simulink model "AirplaneSimModel_Trim"  (R2025b)
settings: Solver=ode1  StartTime=0.0  StopTime=1  RelTol=1e-3
model workspace (MAT data in the model file):
  initial_input_in_model_workspace = [0 0.010416783094 0.861959012587 0.2094 -0.018208861967 0.815245721637]
  initial_state_in_model_workspace.time = 0
  initial_state_in_model_workspace.signals(1).values = [0 0 0]
  initial_state_in_model_workspace.signals(1).dimensions = 3
  initial_state_in_model_workspace.signals(1).label = 'CSTATE'
  initial_state_in_model_workspace.signals(1).blockName = 'AirplaneSimModel_Trim/Conventional Airplane,
    | single engine/State equations
    | (Quaternions)/s__g'
  initial_state_in_model_workspace.signals(1).stateName = 'position'
  initial_state_in_model_workspace.signals(1).inReferencedModel = 0
  initial_state_in_model_workspace.signals(1).sampleTime = [0 0]
  initial_state_in_model_workspace.signals(2).values = [0.9988 0 -0.125422444495 0]
  initial_state_in_model_workspace.signals(2).dimensions = 4
  initial_state_in_model_workspace.signals(2).label = 'CSTATE'
  initial_state_in_model_workspace.signals(2).blockName = 'AirplaneSimModel_Trim/Conventional Airplane,
    | single engine/State equations
    | (Quaternions)/q_bg'
  initial_state_in_model_workspace.signals(2).stateName = 'quaternion'
  initial_state_in_model_workspace.signals(2).inReferencedModel = 0
  initial_state_in_model_workspace.signals(2).sampleTime = [0 0]
  initial_state_in_model_workspace.signals(3).values = 797.872042942
  initial_state_in_model_workspace.signals(3).dimensions = 1
  initial_state_in_model_workspace.signals(3).label = 'CSTATE'
  initial_state_in_model_workspace.signals(3).blockName = 'AirplaneSimModel_Trim/Conventional Airplane,
    | single engine/Actuators/Integrator'
  initial_state_in_model_workspace.signals(3).stateName = 'motor_speed'
  initial_state_in_model_workspace.signals(3).inReferencedModel = 0
  initial_state_in_model_workspace.signals(3).sampleTime = [0 0]
  initial_state_in_model_workspace.signals(4).values = 0.0767491085272
  initial_state_in_model_workspace.signals(4).dimensions = 1
  initial_state_in_model_workspace.signals(4).label = 'CSTATE'
  initial_state_in_model_workspace.signals(4).blockName = 'AirplaneSimModel_Trim/Conventional Airplane,
    | single engine/Actuators/Nonlinear Second-Order Actuator
    | (elevons)/A'
  initial_state_in_model_workspace.signals(4).stateName = 'A'
  initial_state_in_model_workspace.signals(4).inReferencedModel = 0
  initial_state_in_model_workspace.signals(4).sampleTime = [0 0]
  initial_state_in_model_workspace.signals(5).values = 0.0434586983747
  initial_state_in_model_workspace.signals(5).dimensions = 1
  initial_state_in_model_workspace.signals(5).label = 'CSTATE'
  initial_state_in_model_workspace.signals(5).blockName = 'AirplaneSimModel_Trim/Conventional Airplane,
    | single engine/Actuators/Nonlinear Second-Order Actuator
    | (htpTrim)/A'
  initial_state_in_model_workspace.signals(5).stateName = 'A'
  initial_state_in_model_workspace.signals(5).inReferencedModel = 0
  initial_state_in_model_workspace.signals(5).sampleTime = [0 0]
  initial_state_in_model_workspace.signals(6).values = [0.426323238582 0.426323238582 0.416142037484 0.416142037484]
  initial_state_in_model_workspace.signals(6).dimensions = 4
  initial_state_in_model_workspace.signals(6).label = 'CSTATE'
  initial_state_in_model_workspace.signals(6).blockName = 'AirplaneSimModel_Trim/Conventional Airplane,
    | single engine/Actuators/Nonlinear Second-Order Actuator
    | (ailerons)/A'
  initial_state_in_model_workspace.signals(6).stateName = 'A'
  initial_state_in_model_workspace.signals(6).inReferencedModel = 0
  initial_state_in_model_workspace.signals(6).sampleTime = [0 0]
  initial_state_in_model_workspace.signals(7).values = -0.00858072404785
  initial_state_in_model_workspace.signals(7).dimensions = 1
  initial_state_in_model_workspace.signals(7).label = 'CSTATE'
  initial_state_in_model_workspace.signals(7).blockName = 'AirplaneSimModel_Trim/Conventional Airplane,
    | single engine/Actuators/Nonlinear Second-Order Actuator
    | (rudder)/A'
  initial_state_in_model_workspace.signals(7).stateName = 'A'
  initial_state_in_model_workspace.signals(7).inReferencedModel = 0
  initial_state_in_model_workspace.signals(7).sampleTime = [0 0]
  initial_state_in_model_workspace.signals(8).values = [16.4721900378 0 -4.20320774642]
  initial_state_in_model_workspace.signals(8).dimensions = 3
  initial_state_in_model_workspace.signals(8).label = 'CSTATE'
  initial_state_in_model_workspace.signals(8).blockName = 'AirplaneSimModel_Trim/Conventional Airplane,
    | single engine/State equations
    | (Quaternions)/V__Kb'
  initial_state_in_model_workspace.signals(8).stateName = 'velocity'
  initial_state_in_model_workspace.signals(8).inReferencedModel = 0
  initial_state_in_model_workspace.signals(8).sampleTime = [0 0]
  initial_state_in_model_workspace.signals(9).values = [0 0 0]
  initial_state_in_model_workspace.signals(9).dimensions = 3
  initial_state_in_model_workspace.signals(9).label = 'CSTATE'
  initial_state_in_model_workspace.signals(9).blockName = 'AirplaneSimModel_Trim/Conventional Airplane,
    | single engine/State equations
    | (Quaternions)/rates'
  initial_state_in_model_workspace.signals(9).stateName = 'rates'
  initial_state_in_model_workspace.signals(9).inReferencedModel = 0
  initial_state_in_model_workspace.signals(9).sampleTime = [0 0]
  initial_state_in_model_workspace.signals(10).values = 1.2134149432
  initial_state_in_model_workspace.signals(10).dimensions = 1
  initial_state_in_model_workspace.signals(10).label = 'CSTATE'
  initial_state_in_model_workspace.signals(10).blockName = 'AirplaneSimModel_Trim/Conventional Airplane,
    | single engine/Conventional Airplane Aerodynamics
    | simple/Downwash/Delay/Integrator'
  initial_state_in_model_workspace.signals(10).stateName = ''
  initial_state_in_model_workspace.signals(10).inReferencedModel = 0
  initial_state_in_model_workspace.signals(10).sampleTime = [0 0]
  initial_state_in_model_workspace.signals(11).values = [0 0 0 0]
  initial_state_in_model_workspace.signals(11).dimensions = 4
  initial_state_in_model_workspace.signals(11).label = 'CSTATE'
  initial_state_in_model_workspace.signals(11).blockName = 'AirplaneSimModel_Trim/Conventional Airplane,
    | single engine/Actuators/Nonlinear Second-Order Actuator
    | (ailerons)/dot_A'
  initial_state_in_model_workspace.signals(11).stateName = 'dot_A'
  initial_state_in_model_workspace.signals(11).inReferencedModel = 0
  initial_state_in_model_workspace.signals(11).sampleTime = [0 0]
  initial_state_in_model_workspace.signals(12).values = 0
  initial_state_in_model_workspace.signals(12).dimensions = 1
  initial_state_in_model_workspace.signals(12).label = 'CSTATE'
  initial_state_in_model_workspace.signals(12).blockName = 'AirplaneSimModel_Trim/Conventional Airplane,
    | single engine/Actuators/Nonlinear Second-Order Actuator
    | (elevons)/dot_A'
  initial_state_in_model_workspace.signals(12).stateName = 'dot_A'
  initial_state_in_model_workspace.signals(12).inReferencedModel = 0
  initial_state_in_model_workspace.signals(12).sampleTime = [0 0]
  initial_state_in_model_workspace.signals(13).values = 0
  initial_state_in_model_workspace.signals(13).dimensions = 1
  initial_state_in_model_workspace.signals(13).label = 'CSTATE'
  initial_state_in_model_workspace.signals(13).blockName = 'AirplaneSimModel_Trim/Conventional Airplane,
    | single engine/Actuators/Nonlinear Second-Order Actuator
    | (htpTrim)/dot_A'
  initial_state_in_model_workspace.signals(13).stateName = 'dot_A'
  initial_state_in_model_workspace.signals(13).inReferencedModel = 0
  initial_state_in_model_workspace.signals(13).sampleTime = [0 0]
  initial_state_in_model_workspace.signals(14).values = 0
  initial_state_in_model_workspace.signals(14).dimensions = 1
  initial_state_in_model_workspace.signals(14).label = 'CSTATE'
  initial_state_in_model_workspace.signals(14).blockName = 'AirplaneSimModel_Trim/Conventional Airplane,
    | single engine/Actuators/Nonlinear Second-Order Actuator
    | (rudder)/dot_A'
  initial_state_in_model_workspace.signals(14).stateName = 'dot_A'
  initial_state_in_model_workspace.signals(14).inReferencedModel = 0
  initial_state_in_model_workspace.signals(14).sampleTime = [0 0]
  initial_state_in_model_workspace.signals(15).values = [0 0 0 0]
  initial_state_in_model_workspace.signals(15).dimensions = 4
  initial_state_in_model_workspace.signals(15).label = 'CSTATE'
  initial_state_in_model_workspace.signals(15).blockName = 'AirplaneSimModel_Trim/Conventional Airplane,
    | single engine/Conventional Airplane Aerodynamics
    | simple/wing 2 point aerodynamics
    | (vertical tailplane, vtp)/Simple Wing Aerodynamics/Unsteady lift/Unsteady lift/Integrator'
  initial_state_in_model_workspace.signals(15).stateName = ''
  initial_state_in_model_workspace.signals(15).inReferencedModel = 0
  initial_state_in_model_workspace.signals(15).sampleTime = [0 0]
  initial_state_in_model_workspace.signals(16).values = [0 0 0 0]
  initial_state_in_model_workspace.signals(16).dimensions = 4
  initial_state_in_model_workspace.signals(16).label = 'CSTATE'
  initial_state_in_model_workspace.signals(16).blockName = 'AirplaneSimModel_Trim/Conventional Airplane,
    | single engine/Conventional Airplane Aerodynamics
    | simple/wing 2 point aerodynamics
    | (vertical tailplane, vtp)/Simple Wing Aerodynamics/Unsteady lift/Unsteady lift/Integrator1'
  initial_state_in_model_workspace.signals(16).stateName = ''
  initial_state_in_model_workspace.signals(16).inReferencedModel = 0
  initial_state_in_model_workspace.signals(16).sampleTime = [0 0]
  initial_state_in_model_workspace.signals(17).values = [0 0 0 0]
  initial_state_in_model_workspace.signals(17).dimensions = 4
  initial_state_in_model_workspace.signals(17).label = 'CSTATE'
  initial_state_in_model_workspace.signals(17).blockName = 'AirplaneSimModel_Trim/Conventional Airplane,
    | single engine/Conventional Airplane Aerodynamics
    | simple/wing 2 point aerodynamics
    | (main wing)/Simple Wing Aerodynamics/Unsteady lift/Unsteady lift/Integrator'
  initial_state_in_model_workspace.signals(17).stateName = ''
  initial_state_in_model_workspace.signals(17).inReferencedModel = 0
  initial_state_in_model_workspace.signals(17).sampleTime = [0 0]
  initial_state_in_model_workspace.signals(18).values = [0 0 0 0 0 0 0 0]
  initial_state_in_model_workspace.signals(18).dimensions = 8
  initial_state_in_model_workspace.signals(18).label = 'CSTATE'
  initial_state_in_model_workspace.signals(18).blockName = 'AirplaneSimModel_Trim/Conventional Airplane,
    | single engine/Conventional Airplane Aerodynamics
    | simple/wing 2 point aerodynamics
    | (main wing)/Simple Wing Aerodynamics/Unsteady lift/Unsteady lift/Integrator1'
  initial_state_in_model_workspace.signals(18).stateName = ''
  initial_state_in_model_workspace.signals(18).inReferencedModel = 0
  initial_state_in_model_workspace.signals(18).sampleTime = [0 0]
  initial_state_in_model_workspace.signals(19).values = [0 0 0 0]
  initial_state_in_model_workspace.signals(19).dimensions = 4
  initial_state_in_model_workspace.signals(19).label = 'CSTATE'
  initial_state_in_model_workspace.signals(19).blockName = 'AirplaneSimModel_Trim/Conventional Airplane,
    | single engine/Conventional Airplane Aerodynamics
    | simple/wing 2 point aerodynamics
    | (horizontal tailplane, htp)/Simple Wing Aerodynamics/Unsteady lift/Unsteady lift/Integrator'
  initial_state_in_model_workspace.signals(19).stateName = ''
  initial_state_in_model_workspace.signals(19).inReferencedModel = 0
  initial_state_in_model_workspace.signals(19).sampleTime = [0 0]
  initial_state_in_model_workspace.signals(20).values = [0 0 0 0]
  initial_state_in_model_workspace.signals(20).dimensions = 4
  initial_state_in_model_workspace.signals(20).label = 'CSTATE'
  initial_state_in_model_workspace.signals(20).blockName = 'AirplaneSimModel_Trim/Conventional Airplane,
    | single engine/Conventional Airplane Aerodynamics
    | simple/wing 2 point aerodynamics
    | (horizontal tailplane, htp)/Simple Wing Aerodynamics/Unsteady lift/Unsteady lift/Integrator1'
  initial_state_in_model_workspace.signals(20).stateName = ''
  initial_state_in_model_workspace.signals(20).inReferencedModel = 0
  initial_state_in_model_workspace.signals(20).sampleTime = [0 0]
undefined symbols (not defined in the file): aileron_left, aileron_right, airplane, alt_ground, atmosphere, elevator, envir, g, htp_trim, rudder, throttle, wind
libraries: unit_conversions_lib x6, flightgear_visualization_lib x2, conventional_airplane_single_engine_lib x1, atmosphere_lib x1, simulink_extras x1
settings Model: Creator=aroan  LastModifiedBy=aroan
settings DataIOCC: ExternalInput=initial_input_in_model_workspace  InitialState=initial_state_in_model_workspace  SaveFormat=Structure
settings DebuggingCC: InitInArrayFormatMsg=none

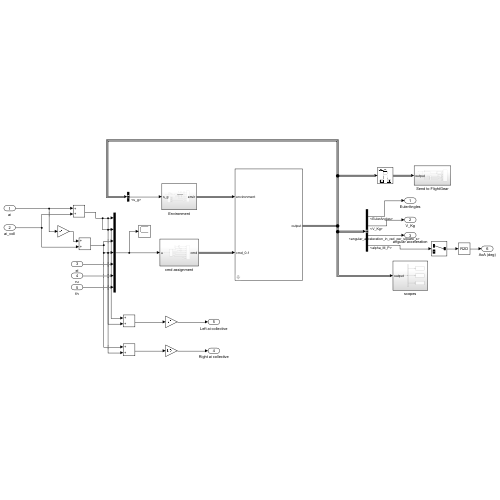
[thumbnail: Simulink's stored preview of the top-level diagram]
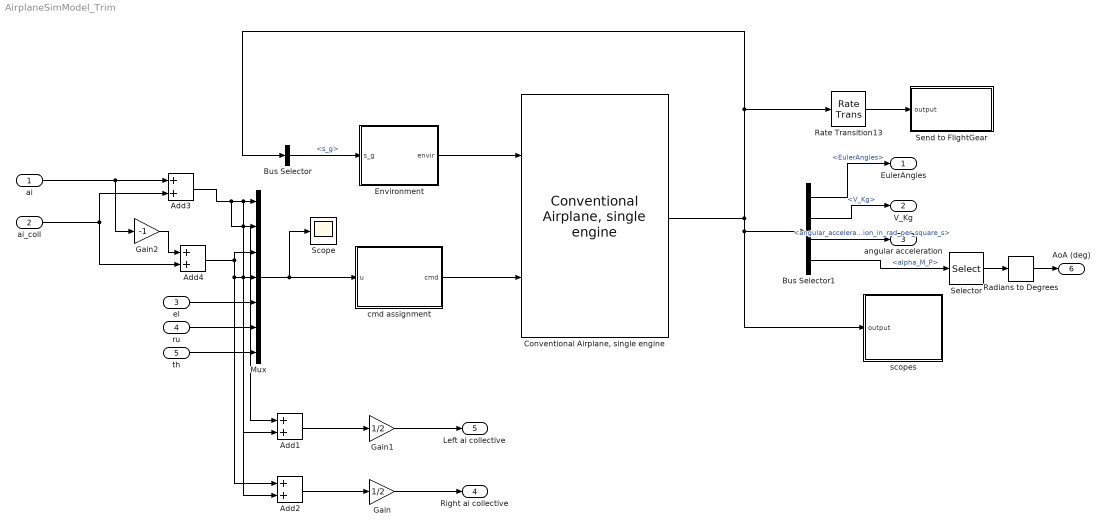
== system AirplaneSimModel_Trim ==
  ai : Inport
  ai_coll : Inport  Port=2
  el : Inport  Port=3
  ru : Inport  Port=4
  th : Inport  Port=5
  Add{1..4} (4 alike) : Sum
  Bus Selector : BusSelector  OutputSignals=rigidBodyBus.s_g
  Bus Selector1 : BusSelector  OutputSignals=rigidBodyBus.EulerAngles,rigidBodyBus.V_Kg,actuatorBus.motorBus.angular_acceleration_in_rad_per_square_s,aeroBus.aeroMainWing.aeroAxes.alpha_M_P
  "Conventional Airplane, single engine" : conventional_airplane_single_engine_lib/Conventional Airplane, single engine  airplane=airplane
      settings: SourceProductName=Conventional Airplane Single Engine
  Environment : Subsystem
  Gain : Gain  Gain=1/2
  Gain1 : Gain  Gain=1/2
  Gain2 : Gain  Gain=-1
  Mux : Mux  Inputs=7
  Radians to Degrees : simulink_extras/Transformations/Radians to Degrees
  Rate Transition13 : RateTransition  OutPortSampleTime=1/50
  Scope : Scope
      settings: ActiveDisplayYMinimum=-0.046898447828128756  ActiveDisplayYMaximum=0.048947358411132957
  Selector : Selector  InputPortWidth=2  IndexOptions=Index vector (dialog)  Indices=1  OutputSizes=1
  Send to FlightGear : Subsystem
  cmd assignment : Subsystem
  scopes : Subsystem
  EulerAngles : Outport
  V_Kg : Outport  Port=2
  angular acceleration : Outport  Port=3
  Right ai collective : Outport  Port=4
  Left ai collective : Outport  Port=5
  AoA (deg) : Outport  Port=6
  wires:
  "Conventional Airplane, single engine"/1 -> Bus Selector1/1, scopes/1(output), Rate Transition13/1, Bus Selector/1
  cmd assignment/1(cmd) -> "Conventional Airplane, single engine"/2
  Rate Transition13/1 -> Send to FlightGear/1(output)
  ru/1 -> Mux/6
  Bus Selector/1 -> Environment/1(s_g)  "<s_g>"
  th/1 -> Mux/7
  Bus Selector1/1 -> EulerAngles/1  "<EulerAngles>"
  Bus Selector1/2 -> V_Kg/1  "<V_Kg>"
  Mux/1 -> Scope/1, cmd assignment/1(u)
  Environment/1(envir) -> "Conventional Airplane, single engine"/1
  Bus Selector1/3 -> angular acceleration/1  "<angular_acceleration_in_rad_per_square_s>"
  el/1 -> Mux/5
  Add1/1 -> Gain1/1
  Add2/1 -> Gain/1
  Gain/1 -> Right ai collective/1
  Gain1/1 -> Left ai collective/1
  Add4/1 -> Add2/1, Add2/2, Mux/4, Mux/3
  Gain2/1 -> Add4/1
  ai/1 -> Gain2/1, Add3/1
  ai_coll/1 -> Add3/2, Add4/2
  Add3/1 -> Add1/2, Mux/1, Add1/1, Mux/2
  Bus Selector1/4 -> Selector/1  "<alpha_M_P>"
  Selector/1 -> Radians to Degrees/1
  Radians to Degrees/1 -> AoA (deg)/1

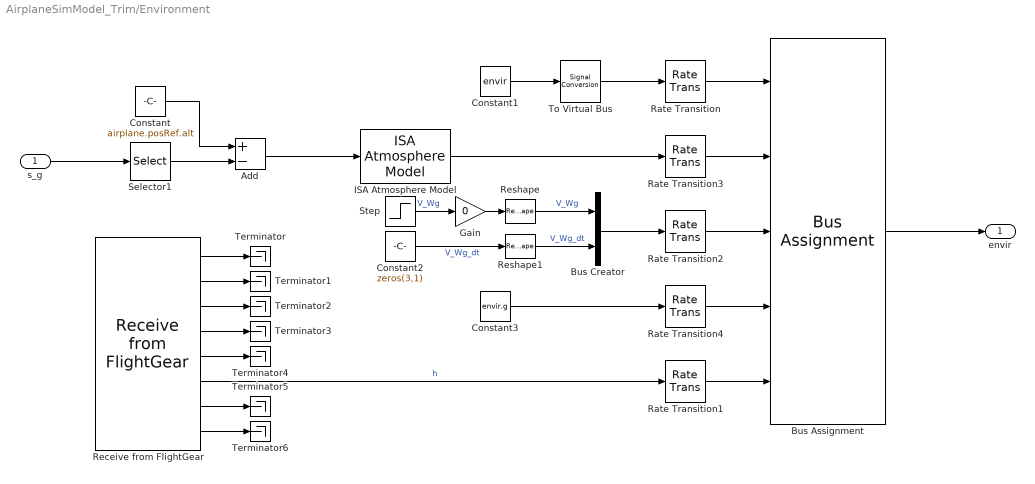
== system AirplaneSimModel_Trim/Environment ==
  s_g : Inport
  Add : Sum  Inputs=+-
  Bus Assignment : BusAssignment  AssignedSignals=atmosphere,wind,g,alt_ground
  Bus Creator : BusCreator  Inputs=2
  Constant : Constant  Value=airplane.posRef.alt
  Constant1 : Constant  Value=envir  OutDataTypeStr=Bus: envirBus
  Constant2 : Constant  Value=zeros(3,1)
  Constant3 : Constant  Value=envir.g
  Gain : Gain  Gain=0
  ISA Atmosphere Model : atmosphere_lib/ISA Atmosphere Model
      settings: SourceProductName=Atmosphere
  Rate Transition{,1..4} (5 alike) : RateTransition
  Receive from FlightGear : flightgear_visualization_lib/Receive from FlightGear  ip_address='127.0.0.1'  ip_port=5503  sample_time=1/40  blocking_time=0  is_aerocntrl=off  is_engine=off  is_fuel=off  is_land=off  is_avionics=off  is_envir=on
      settings: SourceProductName=FlightGear visualization
  Reshape : Reshape  OutputDimensionality=Column vector (2-D)
  Reshape1 : Reshape  OutputDimensionality=Column vector (2-D)
  Selector1 : Selector  InputPortWidth=3  IndexOptions=Index vector (dialog)  Indices=3  OutputSizes=1
  Step : Step  Time=3  After=[0;9;0]  SampleTime=0
  Terminator{,1..6} (7 alike) : Terminator
  To Virtual Bus : SignalConversion  ConversionOutput=Virtual bus  OverrideOpt=off
  envir : Outport  VectorParamsAs1DForOutWhenUnconnected=off
  wires:
  Rate Transition2/1 -> Bus Assignment/3
  Rate Transition3/1 -> Bus Assignment/2
  Bus Assignment/1 -> envir/1
  Rate Transition/1 -> Bus Assignment/1
  ISA Atmosphere Model/1 -> Rate Transition3/1
  Step/1 -> Gain/1  "V_Wg"
  Rate Transition1/1 -> Bus Assignment/5
  Constant1/1 -> To Virtual Bus/1
  s_g/1 -> Selector1/1
  Bus Creator/1 -> Rate Transition2/1
  Constant2/1 -> Reshape1/1  "V_Wg_dt"
  Rate Transition4/1 -> Bus Assignment/4
  Constant3/1 -> Rate Transition4/1
  Gain/1 -> Reshape/1
  Constant/1 -> Add/1
  Add/1 -> ISA Atmosphere Model/1
  Selector1/1 -> Add/2
  To Virtual Bus/1 -> Rate Transition/1
  Reshape/1 -> Bus Creator/1  "V_Wg"
  Reshape1/1 -> Bus Creator/2  "V_Wg_dt"
  Receive from FlightGear/3 -> Terminator2/1
  Receive from FlightGear/1 -> Terminator/1
  Receive from FlightGear/6 -> Rate Transition1/1  "h"
  Receive from FlightGear/2 -> Terminator1/1
  Receive from FlightGear/5 -> Terminator4/1
  Receive from FlightGear/7 -> Terminator5/1
  Receive from FlightGear/4 -> Terminator3/1
  Receive from FlightGear/8 -> Terminator6/1

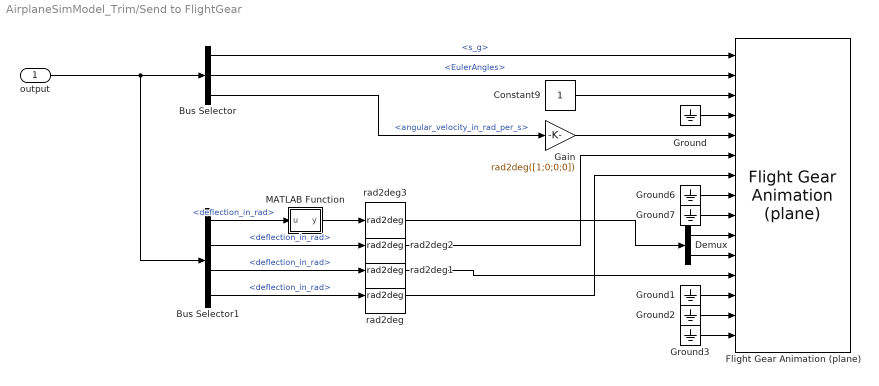
== system AirplaneSimModel_Trim/Send to FlightGear ==
  output : Inport
  Bus Selector : BusSelector  OutputSignals=rigidBodyBus.s_g,rigidBodyBus.EulerAngles,actuatorBus.motorBus.angular_velocity_in_rad_per_s
  Bus Selector1 : BusSelector  OutputSignals=actuatorBus.aileronsBus.deflection_in_rad,actuatorBus.elevatorBus.deflection_in_rad,actuatorBus.rudderBus.deflection_in_rad,actuatorBus.htpTrimBus.deflection_in_rad
  Constant9 : Constant
  Demux : Demux  Outputs=2
  Flight Gear Animation (plane) : flightgear_visualization_lib/Flight Gear Animation (plane)  inital_lat=airplane.posRef.lat  inital_long=airplane.posRef.lon  inital_height=airplane.posRef.alt  remoteURL='127.0.0.1'  remotePort=5502
      settings: SourceProductName=FlightGear visualization
  Gain : Gain  Gain=rad2deg([1;0;0;0])
  Ground{,1..3,6..7} (6 alike) : Ground
  MATLAB Function : MATLAB Function  TreatAsAtomicUnit=on
  rad2deg{,1..3} (4 alike) : unit_conversions_lib/rad2deg
      settings: SourceProductName=Unit Conversions
  wires:
  Bus Selector/1 -> Flight Gear Animation (plane)/1  "<s_g>"
  Bus Selector/2 -> Flight Gear Animation (plane)/2  "<EulerAngles>"
  Gain/1 -> Flight Gear Animation (plane)/5
  Constant9/1 -> Flight Gear Animation (plane)/3
  Ground/1 -> Flight Gear Animation (plane)/4
  Ground1/1 -> Flight Gear Animation (plane)/13
  Ground2/1 -> Flight Gear Animation (plane)/14
  Ground3/1 -> Flight Gear Animation (plane)/15
  output/1 -> Bus Selector1/1, Bus Selector/1
  Bus Selector/3 -> Gain/1  "<angular_velocity_in_rad_per_s>"
  Bus Selector1/2 -> rad2deg2/1  "<deflection_in_rad>"
  Bus Selector1/4 -> rad2deg/1  "<deflection_in_rad>"
  Ground6/1 -> Flight Gear Animation (plane)/8
  Ground7/1 -> Flight Gear Animation (plane)/9
  Bus Selector1/3 -> rad2deg1/1  "<deflection_in_rad>"
  Bus Selector1/1 -> MATLAB Function/1(u)  "<deflection_in_rad>"
  Demux/1 -> Flight Gear Animation (plane)/10
  Demux/2 -> Flight Gear Animation (plane)/11
  rad2deg/1 -> Flight Gear Animation (plane)/7
  rad2deg1/1 -> Flight Gear Animation (plane)/12
  rad2deg2/1 -> Flight Gear Animation (plane)/6
  rad2deg3/1 -> Demux/1
  MATLAB Function/1(y) -> rad2deg3/1

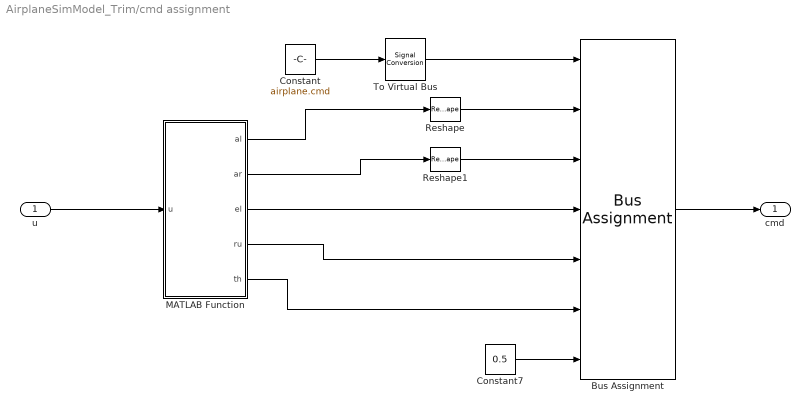
== system AirplaneSimModel_Trim/cmd assignment ==
  u : Inport
  Bus Assignment : BusAssignment  AssignedSignals=aileron_left,aileron_right,elevator,rudder,throttle,htp_trim
  Constant : Constant  Value=airplane.cmd  OutDataTypeStr=Bus: cmdBus
  Constant7 : Constant  Value=0.5
  MATLAB Function : MATLAB Function  TreatAsAtomicUnit=on
  Reshape : Reshape  OutputDimensionality=Row vector (2-D)
  Reshape1 : Reshape  OutputDimensionality=Row vector (2-D)
  To Virtual Bus : SignalConversion  ConversionOutput=Virtual bus  OverrideOpt=off
  cmd : Outport  VectorParamsAs1DForOutWhenUnconnected=off
  wires:
  Constant/1 -> To Virtual Bus/1
  Bus Assignment/1 -> cmd/1
  Constant7/1 -> Bus Assignment/7
  u/1 -> MATLAB Function/1(u)
  MATLAB Function/4(ru) -> Bus Assignment/5
  To Virtual Bus/1 -> Bus Assignment/1
  MATLAB Function/1(al) -> Reshape/1
  MATLAB Function/2(ar) -> Reshape1/1
  MATLAB Function/5(th) -> Bus Assignment/6
  Reshape/1 -> Bus Assignment/2
  Reshape1/1 -> Bus Assignment/3
  MATLAB Function/3(el) -> Bus Assignment/4

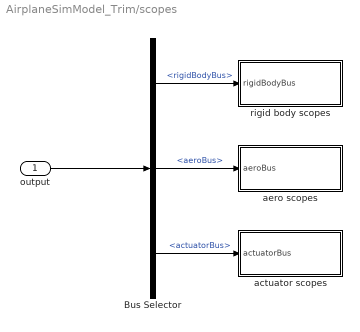
== system AirplaneSimModel_Trim/scopes ==
  output : Inport
  Bus Selector : BusSelector  OutputSignals=rigidBodyBus,aeroBus,actuatorBus
  actuator scopes : Subsystem
  aero scopes : Subsystem
  rigid body scopes : Subsystem
  wires:
  Bus Selector/1 -> rigid body scopes/1(rigidBodyBus)  "<rigidBodyBus>"
  Bus Selector/2 -> aero scopes/1(aeroBus)  "<aeroBus>"
  output/1 -> Bus Selector/1
  Bus Selector/3 -> actuator scopes/1(actuatorBus)  "<actuatorBus>"

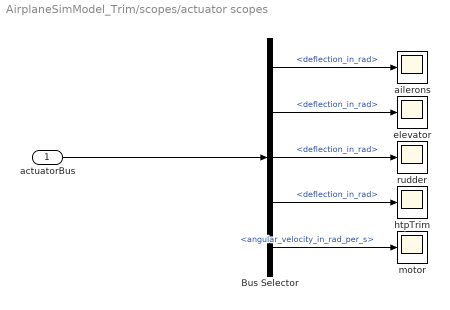
== system AirplaneSimModel_Trim/scopes/actuator scopes ==
  actuatorBus : Inport
  Bus Selector : BusSelector  OutputSignals=aileronsBus.deflection_in_rad,elevatorBus.deflection_in_rad,rudderBus.deflection_in_rad,htpTrimBus.deflection_in_rad,motorBus.angular_velocity_in_rad_per_s
  ailerons : Scope
      settings: ActiveDisplayYMinimum=-0.3126299117513805  ActiveDisplayYMaximum=-0.28991866074071437
  elevator : Scope
      settings: ActiveDisplayYMinimum=0.0083259571459404855  ActiveDisplayYMaximum=0.028325957145940488  DataLoggingVariableName=ScopeData2
  htpTrim : Scope
      settings: ActiveDisplayYMinimum=-1  ActiveDisplayYMaximum=1  DataLoggingVariableName=ScopeData4
  motor : Scope
      settings: ActiveDisplayYMinimum=736.85007954344474  ActiveDisplayYMaximum=1052.4986742759011  DataLoggingVariableName=ScopeData5
  rudder : Scope
      settings: ActiveDisplayYMinimum=0.0072112312119573625  ActiveDisplayYMaximum=0.0092112312119574588  DataLoggingVariableName=ScopeData3
  wires:
  actuatorBus/1 -> Bus Selector/1
  Bus Selector/1 -> ailerons/1  "<deflection_in_rad>"
  Bus Selector/2 -> elevator/1  "<deflection_in_rad>"
  Bus Selector/3 -> rudder/1  "<deflection_in_rad>"
  Bus Selector/4 -> htpTrim/1  "<deflection_in_rad>"
  Bus Selector/5 -> motor/1  "<angular_velocity_in_rad_per_s>"

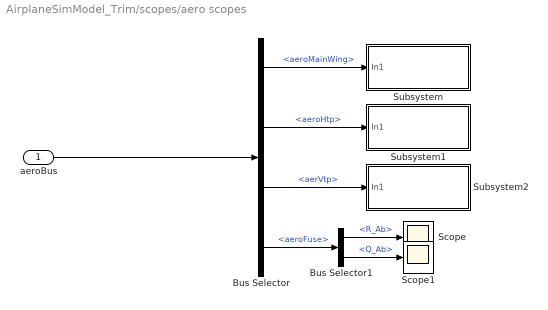
== system AirplaneSimModel_Trim/scopes/aero scopes ==
  aeroBus : Inport
  Bus Selector : BusSelector  OutputSignals=aeroMainWing,aeroHtp,aerVtp,aeroFuse
  Bus Selector1 : BusSelector  OutputSignals=R_Ab,Q_Ab
  Scope : Scope
      settings: ActiveDisplayYMinimum=-4.29896  ActiveDisplayYMaximum=2.72976  DataLoggingVariableName=ScopeData8
  Scope1 : Scope
      settings: ActiveDisplayYMinimum=-0.0040360824438954359  ActiveDisplayYMaximum=0.0038282429936045653  DataLoggingVariableName=ScopeData9
  Subsystem : Subsystem
  Subsystem1 : Subsystem
  Subsystem2 : Subsystem
  wires:
  aeroBus/1 -> Bus Selector/1
  Bus Selector/1 -> Subsystem/1(In1)  "<aeroMainWing>"
  Bus Selector/2 -> Subsystem1/1(In1)  "<aeroHtp>"
  Bus Selector/3 -> Subsystem2/1(In1)  "<aerVtp>"
  Bus Selector/4 -> Bus Selector1/1  "<aeroFuse>"
  Bus Selector1/1 -> Scope/1  "<R_Ab>"
  Bus Selector1/2 -> Scope1/1  "<Q_Ab>"

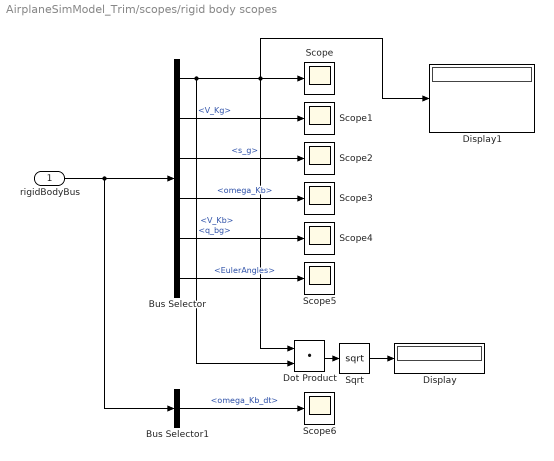
== system AirplaneSimModel_Trim/scopes/rigid body scopes ==
  rigidBodyBus : Inport
  Bus Selector : BusSelector  OutputSignals=V_Kb,V_Kg,s_g,omega_Kb,q_bg,EulerAngles
  Bus Selector1 : BusSelector  OutputSignals=omega_Kb_dt
  Display : Display
  Display1 : Display
  Dot Product : DotProduct  OutDataTypeStr=Inherit: Inherit via internal rule
  Scope{,1..6} (7 alike) : Scope
      Scope settings: ActiveDisplayYMinimum=-8.2513600344443958  ActiveDisplayYMaximum=8.5989912895395726
      Scope1 settings: ActiveDisplayYMinimum=-28.92052  ActiveDisplayYMaximum=41.40763  DataLoggingVariableName=ScopeData2
      Scope2 settings: ActiveDisplayYMinimum=-4.8033  ActiveDisplayYMaximum=9.26764  DataLoggingVariableName=s_g
      Scope3 settings: ActiveDisplayYMinimum=-1.2256864098708227  ActiveDisplayYMaximum=0.58304887183806975  DataLoggingVariableName=ScopeData4
      Scope4 settings: ActiveDisplayYMinimum=-1.2621554909283943  ActiveDisplayYMaximum=1.2639133990800713  DataLoggingVariableName=ScopeData5
      Scope5 settings: ActiveDisplayYMinimum=-3.9260363827841269  ActiveDisplayYMaximum=3.9265382890596952  DataLoggingVariableName=ScopeData6
      Scope6 settings: ActiveDisplayYMinimum=-35.25832  ActiveDisplayYMaximum=13.8699  DataLoggingVariableName=ScopeData6
  Sqrt : Sqrt
  wires:
  rigidBodyBus/1 -> Bus Selector1/1, Bus Selector/1
  Bus Selector/1 -> Dot Product/1, Scope/1, Display1/1, Dot Product/2  "<V_Kb>"
  Bus Selector/2 -> Scope1/1  "<V_Kg>"
  Bus Selector/3 -> Scope2/1  "<s_g>"
  Bus Selector/4 -> Scope3/1  "<omega_Kb>"
  Bus Selector/5 -> Scope4/1  "<q_bg>"
  Bus Selector/6 -> Scope5/1  "<EulerAngles>"
  Dot Product/1 -> Sqrt/1
  Sqrt/1 -> Display/1
  Bus Selector1/1 -> Scope6/1  "<omega_Kb_dt>"

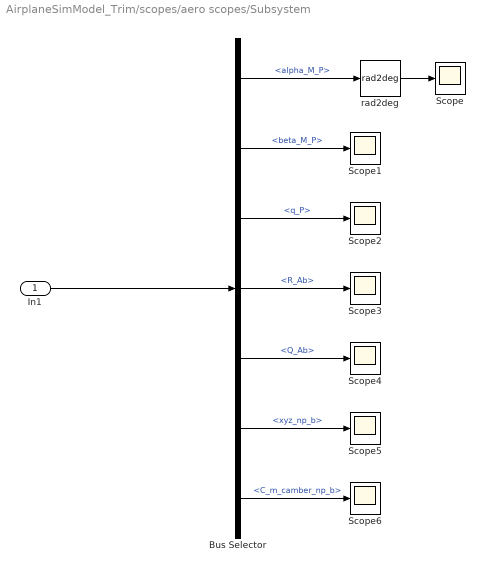
== system AirplaneSimModel_Trim/scopes/aero scopes/Subsystem ==
  In1 : Inport
  Bus Selector : BusSelector  OutputSignals=aeroAxes.alpha_M_P,aeroAxes.beta_M_P,aeroAxes.q_P,dynamicsBody.R_Ab,dynamicsBody.Q_Ab,dynamicsBody.xyz_np_b,dynamicsBody.C_m_camber_np_b
  Scope{,1..6} (7 alike) : Scope
      Scope settings: ActiveDisplayYMinimum=-38.50324  ActiveDisplayYMaximum=61.17596  DataLoggingVariableName=ScopeData3
      Scope1 settings: ActiveDisplayYMinimum=-0.278  ActiveDisplayYMaximum=0.31424  DataLoggingVariableName=ScopeData4
      Scope2 settings: ActiveDisplayYMinimum=-36.957661004904729  ActiveDisplayYMaximum=332.62066571961878  DataLoggingVariableName=ScopeData5
      Scope3 settings: ActiveDisplayYMinimum=-68.5902867146491  ActiveDisplayYMaximum=108.37777420669076  DataLoggingVariableName=ScopeData6
      Scope4 settings: ActiveDisplayYMinimum=-1.14355  ActiveDisplayYMaximum=0.48604  DataLoggingVariableName=ScopeData7
      Scope5 settings: ActiveDisplayYMinimum=-0.7438  ActiveDisplayYMaximum=0.72425  DataLoggingVariableName=ScopeData12
      Scope6 settings: ActiveDisplayYMinimum=-0.11083  ActiveDisplayYMaximum=0.05149
  rad2deg : unit_conversions_lib/rad2deg
      settings: SourceProductName=Unit Conversions
  wires:
  Bus Selector/1 -> rad2deg/1  "<alpha_M_P>"
  Bus Selector/3 -> Scope2/1  "<q_P>"
  Bus Selector/2 -> Scope1/1  "<beta_M_P>"
  Bus Selector/4 -> Scope3/1  "<R_Ab>"
  Bus Selector/5 -> Scope4/1  "<Q_Ab>"
  Bus Selector/6 -> Scope5/1  "<xyz_np_b>"
  Bus Selector/7 -> Scope6/1  "<C_m_camber_np_b>"
  rad2deg/1 -> Scope/1
  In1/1 -> Bus Selector/1

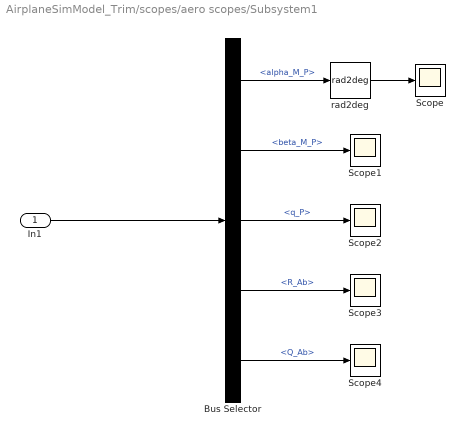
== system AirplaneSimModel_Trim/scopes/aero scopes/Subsystem1 ==
  In1 : Inport
  Bus Selector : BusSelector  OutputSignals=aeroAxes.alpha_M_P,aeroAxes.beta_M_P,aeroAxes.q_P,dynamicsBody.R_Ab,dynamicsBody.Q_Ab
  Scope{,1..4} (5 alike) : Scope
      Scope settings: ActiveDisplayYMinimum=-7.22371  ActiveDisplayYMaximum=26.21378  DataLoggingVariableName=ScopeData3
      Scope1 settings: ActiveDisplayYMinimum=-0.40678  ActiveDisplayYMaximum=0.98354  DataLoggingVariableName=ScopeData4
      Scope2 settings: ActiveDisplayYMinimum=165.0715  ActiveDisplayYMaximum=265.67716  DataLoggingVariableName=ScopeData5
      Scope3 settings: ActiveDisplayYMinimum=-1.25595  ActiveDisplayYMaximum=0.52297  DataLoggingVariableName=ScopeData6
      Scope4 settings: ActiveDisplayYMinimum=-1.24313  ActiveDisplayYMaximum=0.67063  DataLoggingVariableName=ScopeData7
  rad2deg : unit_conversions_lib/rad2deg
      settings: SourceProductName=Unit Conversions
  wires:
  Bus Selector/5 -> Scope4/1  "<Q_Ab>"
  Bus Selector/4 -> Scope3/1  "<R_Ab>"
  Bus Selector/2 -> Scope1/1  "<beta_M_P>"
  Bus Selector/3 -> Scope2/1  "<q_P>"
  Bus Selector/1 -> rad2deg/1  "<alpha_M_P>"
  In1/1 -> Bus Selector/1
  rad2deg/1 -> Scope/1

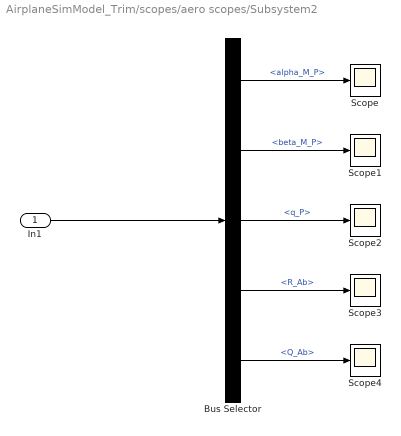
== system AirplaneSimModel_Trim/scopes/aero scopes/Subsystem2 ==
  In1 : Inport
  Bus Selector : BusSelector  OutputSignals=aeroAxes.alpha_M_P,aeroAxes.beta_M_P,aeroAxes.q_P,dynamicsBody.R_Ab,dynamicsBody.Q_Ab
  Scope{,1..4} (5 alike) : Scope
      Scope settings: ActiveDisplayYMinimum=-0.0091  ActiveDisplayYMaximum=0.08194  DataLoggingVariableName=ScopeData3
      Scope1 settings: ActiveDisplayYMinimum=-0.04947  ActiveDisplayYMaximum=0.04829  DataLoggingVariableName=ScopeData4
      Scope2 settings: DataLoggingVariableName=ScopeData5
      Scope3 settings: ActiveDisplayYMinimum=-0.28199  ActiveDisplayYMaximum=0.15437  DataLoggingVariableName=ScopeData6
      Scope4 settings: ActiveDisplayYMinimum=-0.01092  ActiveDisplayYMaximum=0.00318  DataLoggingVariableName=ScopeData7
  wires:
  In1/1 -> Bus Selector/1
  Bus Selector/1 -> Scope/1  "<alpha_M_P>"
  Bus Selector/3 -> Scope2/1  "<q_P>"
  Bus Selector/2 -> Scope1/1  "<beta_M_P>"
  Bus Selector/4 -> Scope3/1  "<R_Ab>"
  Bus Selector/5 -> Scope4/1  "<Q_Ab>"

== matlab function AirplaneSimModel_Trim/cmd assignment/MATLAB Function ==
  data: u input; al output; ar output; el output; ru output; th output
function [al,ar,el,ru,th] = fcn(u)
ai = u(1:end-3) * 0.5 + 0.5;
al = ai(1:end/2);
ar = ai(end/2+1:end);
el = u(end-2) * 0.5 + 0.5;
ru = u(end-1) * 0.5 + 0.5;
th = u(end);
end

== matlab function AirplaneSimModel_Trim/Send to FlightGear/MATLAB Function ==
  data: u input; y output
function y = fcn(u)

y = u([1,end])';
